simulink model "SF5_1_5_jc0701_1"  (R2017a)
settings: Solver=FixedStepDiscrete  StartTime=0.0  StopTime=10.0  RelTol=1e-3  EnableMultiTasking=on
PostLoadFcn:
  | % -------------------------------------------------------------------
  | %  Generated by MATLAB on 10-Feb-2017 13:23:05
  | %  MATLAB version: 9.1.0.441655 (R2016b)
  | % -------------------------------------------------------------------
  | 
  | 
  | diffName = Simulink.Signal;
  | diffName.CoderInfo.StorageClass = 'ExportedGlobal';
  | diffName.CoderInfo.Alias = '';
  | diffName.CoderInfo.Alignment = -1;
  | diffName.Description = '';
  | diffName.DataType = 'auto';
  | diffName.Min = [];
  | diffName.Max = [];
  | diffName.DocUnits = '';
  | diffName.Dimensions = -1;
  | diffName.DimensionsMode = 'auto';
  | diffName.Complexity = 'auto';
  | diffName.SampleTime = -1;
  | diffName.InitialValue = '';
  | 
  | myinput = Simulink.Signal;
  | myinput.CoderInfo.StorageClass = 'ExportedGlobal';
  | myinput.CoderInfo.Alias = '';
  | myinput.CoderInfo.Alignment = -1;
  | myinput.Description = '';
  | myinput.DataType = 'auto';
  | myinput.Min = [];
  | myinput.Max = [];
  | myinput.DocUnits = '';
  | myinput.Dimensions = -1;
  | myinput.DimensionsMode = 'auto';
  | myinput.Complexity = 'auto';
  | myinput.SampleTime = -1;
  | myinput.InitialValue = '';
  | 
  | out = Simulink.Signal;
  | out.CoderInfo.StorageClass = 'ExportedGlobal';
  | out.CoderInfo.Alias = '';
  | out.CoderInfo.Alignment = -1;
  | out.Description = '';
  | out.DataType = 'auto';
  | out.Min = [];
  | out.Max = [];
  | out.DocUnits = '';
  | out.Dimensions = -1;
  | out.DimensionsMode = 'auto';
  | out.Complexity = 'auto';
  | out.SampleTime = -1;
  | out.InitialValue = '';
  | 
  | out2 = Simulink.Signal;
  | out2.CoderInfo.StorageClass = 'ExportedGlobal';
  | out2.CoderInfo.Alias = '';
  | out2.CoderInfo.Alignment = -1;
  | out2.Description = '';
  | out2.DataType = 'auto';
  | out2.Min = [];
  | out2.Max = [];
  | out2.DocUnits = '';
  | out2.Dimensions = -1;
  | out2.DimensionsMode = 'auto';
  | out2.Complexity = 'auto';
  | out2.SampleTime = -1;
  | out2.InitialValue = '';
  | 
  | param = Simulink.Parameter;
  | param.Value = [1 2 3 4 5];
  | param.CoderInfo.StorageClass = 'ExportedGlobal';
  | param.CoderInfo.Alias = '';
  | param.CoderInfo.Alignment = -1;
  | param.Description = '';
  | param.DataType = 'auto';
  | param.Min = [];
  | param.Max = [];
  | param.DocUnits = '';
settings Model: Creator=amyyang  LastModifiedBy=amyyang
settings DataIOCC: LimitDataPoints=on
settings OptimizationCC: DefaultParameterBehavior=Inlined  LifeSpan=1
settings DebuggingCC: AllowSymbolicDim=off  SFUnexpectedBacktrackingDiag=warning  SFNoUnconditionalDefaultTransitionDiag=warning  SFExecutionAtInitializationDiag=none
settings ModelReferenceCC: PropagateSignalLabelsOutOfModel=off
settings RTWCC: SystemTargetFile=ert.tlc  GenCodeOnly=on  TemplateMakefile=ert_default_tmf  Description=Embedded Coder  GenerateReport=on  IncludeHyperlinkInReport=on  LaunchReport=on  GenerateTraceInfo=on  GenerateTraceReport=on  GenerateTraceReportSl=on  GenerateTraceReportSf=on  GenerateTraceReportEml=on
settings CodeAppCC: IgnoreCustomStorageClasses=off
settings ERTTargetCC: MultiwordLength=2048  GenerateSampleERTMain=on  InlinedParameterPlacement=NonHierarchical  ERTCustomFileTemplate=example_file_process.tlc  ConvertIfToSwitch=off  SuppressUnreachableDefaultCases=off
settings ConfigComp: CovMetricSettings=dw  CovHtmlReporting=on  CovSaveCumulativeToWorkspaceVar=on  CovSaveSingleToWorkspaceVar=on  CovExternalEMLEnable=off

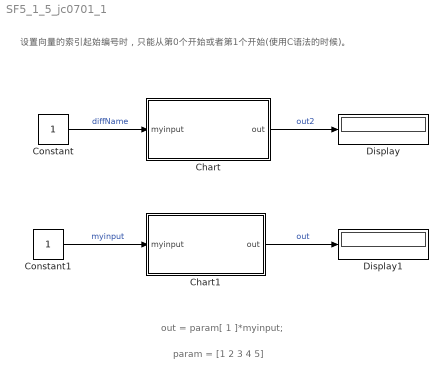
== system SF5_1_5_jc0701_1 ==
  note: param = [1 2 3 4 5]
  note: out = param[ 1 ]*myinput;
  note: 设置向量的索引起始编号时，只能从第0个开始或者第1个开始(使用C语法的时候)。
  Chart : Stateflow chart  TreatAsAtomicUnit=on
  Chart1 : Stateflow chart  TreatAsAtomicUnit=on
  Constant : Constant
  Constant1 : Constant
  Display : Display
  Display1 : Display
  wires:
  Chart/1(out) -> Display/1  "out2"
  Constant/1 -> Chart/1(myinput)  "diffName"
  Chart1/1(out) -> Display1/1  "out"
  Constant1/1 -> Chart1/1(myinput)  "myinput"

== stateflow chart SF5_1_5_jc0701_1/Chart1 ==
  (default) -> (junction 2) : {
      | out = param(1)*myinput;
      | }
  data: out output; myinput input; param parameter

== stateflow chart SF5_1_5_jc0701_1/Chart ==
  (default) -> (junction 2) : {
      | out = param[1]*myinput;
      | }
  data: out output; myinput input; param parameter double size=[1 5]
